simulink subsystem "sensor_distancia"  (R2024a)
settings: Solver=VariableStepAuto  StartTime=0.0  StopTime=10.0  RelTol=1e-3
libraries: arduinolib x2
settings Model: Creator=julia  LastModifiedBy=julia

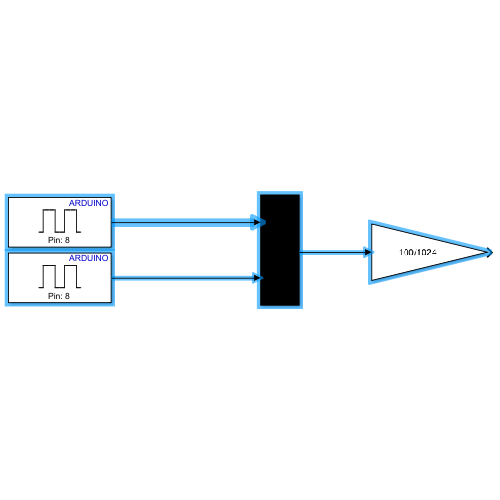
[thumbnail: Simulink's stored preview of the top-level diagram]
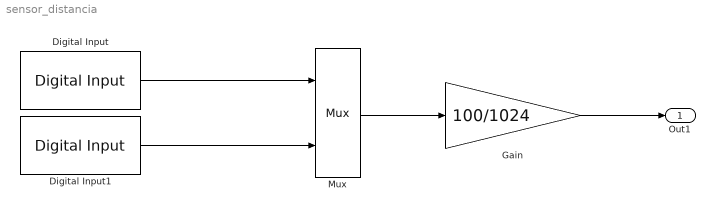
== system sensor_distancia ==
  Digital Input : arduinolib/Digital Input  pinNumber=8  mode=Default  Direction=input  SampleTime=0.1  blockPlatform=arduino
  Digital Input1 : arduinolib/Digital Input  pinNumber=8  mode=Default  Direction=input  SampleTime=0.1  blockPlatform=arduino
  Gain : Gain  Gain=100/1024
  Mux : Mux  Inputs=2
  Out1 : Outport
  wires:
  Mux/1 -> Gain/1
  Digital Input1/1 -> Mux/2
  Digital Input/1 -> Mux/1
  Gain/1 -> Out1/1
